simulink model "simple_rc_circuit_simul"  (R2023a)
settings: Solver=FixedStepAuto  StartTime=0.0  StopTime=10.0  FixedStep=1e-3  RelTol=1e-3
values from neighbouring files (symbols this model uses):
  c = 1e-6    (= 1e-06)    [Simple_rc_circuit.m]
  r = 1000    [Simple_rc_circuit.m]
settings Model: Creator=mazen  LastModifiedBy=mazen

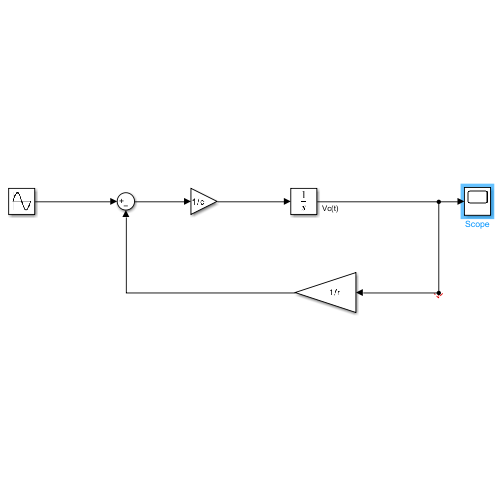
[thumbnail: Simulink's stored preview of the top-level diagram]
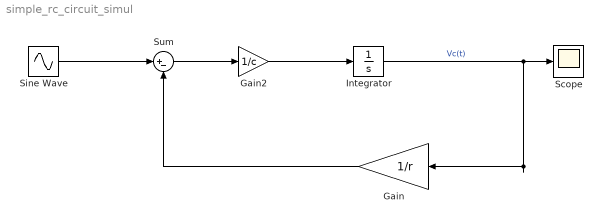
== system simple_rc_circuit_simul ==
  Gain : Gain  Gain=1/r
  Gain2 : Gain  Gain=1/c
  Integrator : Integrator
  Scope : Scope
  Sine Wave : Sin  Amplitude=5  Frequency=1*2*pi  SampleTime=0
  Sum : Sum  Inputs=|+-
  wires:
  Integrator/1 -> Scope/1, Gain/1  "Vc(t)"
  Sum/1 -> Gain2/1
  Sine Wave/1 -> Sum/1
  Gain/1 -> Sum/2
  Gain2/1 -> Integrator/1
